simulink model "sdm_new"  (Simulink 8.1)
settings: Solver=ode45  StartTime=0.0  StopTime=65535  RelTol=1e-3
values from neighbouring files (symbols this model uses):
  sdm_in = FRAC    (= 16385)    [PSD.m]
  w = 17    [PSD.m]
undefined symbols (not defined in the file or in its folder): qunt, qunt1
settings Model: Creator=amr  LastModifiedBy=amr
settings DataIOCC: SignalLoggingSaveFormat=Dataset
settings OptimizationCC: ExpressionDepthLimit=128
settings DebuggingCC: FcnCallInpInsideContextMsg=EnableAllAsError
settings GRTTargetCC: CombineOutputUpdateFcns=on  GRTInterface=off

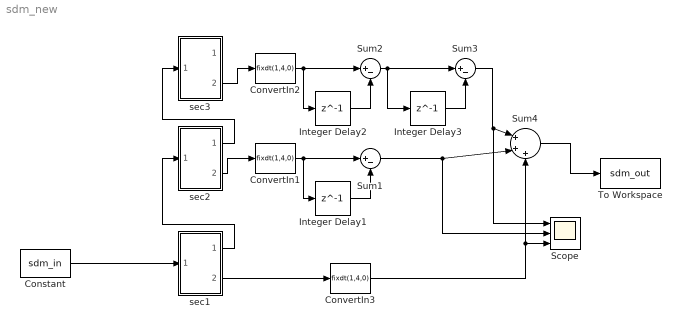
== system sdm_new ==
  Constant : Constant  Value=sdm_in  OutDataTypeStr=fixdt(1,w,0)
  ConvertIn1 : DataTypeConversion  OutDataTypeStr=fixdt(1,4,0)
  ConvertIn2 : DataTypeConversion  OutDataTypeStr=fixdt(1,4,0)
  ConvertIn3 : DataTypeConversion  OutDataTypeStr=fixdt(1,4,0)
  Integer Delay1 : Delay  DelayLength=1  InputProcessing=Inherited
  Integer Delay2 : Delay  DelayLength=1  InputProcessing=Inherited
  Integer Delay3 : Delay  DelayLength=1  InputProcessing=Inherited
  Scope : Scope  NumInputPorts=3
      settings: YMin=-1~-150000~-150000  YMax=1~150000~150000
  Sum1 : Sum  Inputs=|+-  OutDataTypeStr=fixdt(1,4,0)
  Sum2 : Sum  Inputs=|+-  OutDataTypeStr=fixdt(1,4,0)
  Sum3 : Sum  Inputs=|+-  OutDataTypeStr=fixdt(1,4,0)
  Sum4 : Sum  Inputs=|+++  OutDataTypeStr=fixdt(1,4,0)  SaturateOnIntegerOverflow=on
  To Workspace : ToWorkspace  VariableName=sdm_out  SampleTime=-1
  sec1 : Subsystem
  sec2 : Subsystem
  sec3 : Subsystem
  wires:
  Constant/1 -> sec1/1(In1)
  ConvertIn1/1 -> Integer Delay1/1, Sum1/1
  Integer Delay1/1 -> Sum1/2
  sec1/2(Out2) -> ConvertIn3/1
  Sum1/1 -> Scope/2, Sum4/2
  ConvertIn2/1 -> Integer Delay2/1, Sum2/1
  Integer Delay2/1 -> Sum2/2
  Sum2/1 -> Integer Delay3/1, Sum3/1
  Integer Delay3/1 -> Sum3/2
  Sum3/1 -> Scope/1, Sum4/1
  Sum4/1 -> To Workspace/1
  sec2/2(Out2) -> ConvertIn1/1
  sec1/1(Out1) -> sec2/1(In1)
  sec3/2(Out2) -> ConvertIn2/1
  sec2/1(Out1) -> sec3/1(In1)
  ConvertIn3/1 -> Scope/3, Sum4/3

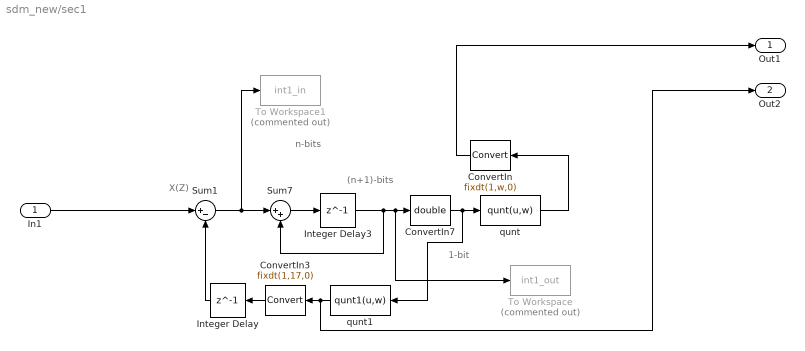
== system sdm_new/sec1 ==
  note: X(Z)
  note: 1-bit
  note: (n+1)-bits
  note: n-bits
  In1 : Inport
  ConvertIn : DataTypeConversion  OutDataTypeStr=fixdt(1,w,0)
  ConvertIn3 : DataTypeConversion  OutDataTypeStr=fixdt(1,17,0)
  ConvertIn7 : DataTypeConversion  OutDataTypeStr=double
  Integer Delay : Delay  DelayLength=1  InputProcessing=Inherited
  Integer Delay3 : Delay  DelayLength=1  InputProcessing=Inherited  SampleTime=1
  Sum1 : Sum  Inputs=|+-  OutDataTypeStr=fixdt(1,w,0)
  Sum7 : Sum  Inputs=|++  AccumDataTypeStr=fixdt(1,w+1,0)  OutDataTypeStr=fixdt(1,w+1,0)
  To Workspace : ToWorkspace  Commented=on  VariableName=int1_out  SampleTime=-1
  To Workspace1 : ToWorkspace  Commented=on  VariableName=int1_in  SampleTime=-1
  qunt : MATLABFcn  MATLABFcn=qunt(u,w)  OutputDimensions=1
  qunt1 : MATLABFcn  MATLABFcn=qunt1(u,w)  OutputDimensions=1
  Out1 : Outport
  Out2 : Outport  Port=2
  wires:
  qunt1/1 -> Out2/1, ConvertIn3/1
  Sum7/1 -> Integer Delay3/1
  qunt/1 -> ConvertIn/1
  ConvertIn7/1 -> qunt1/1, qunt/1
  Integer Delay/1 -> Sum1/2
  ConvertIn/1 -> Out1/1
  ConvertIn3/1 -> Integer Delay/1
  Sum1/1 -> To Workspace1/1, Sum7/1
  In1/1 -> Sum1/1
  Integer Delay3/1 -> To Workspace/1, ConvertIn7/1, Sum7/2

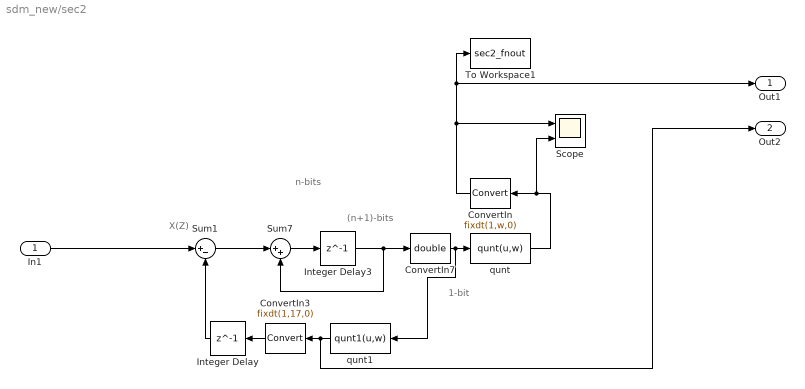
== system sdm_new/sec2 ==
  note: X(Z)
  note: 1-bit
  note: (n+1)-bits
  note: n-bits
  In1 : Inport
  ConvertIn : DataTypeConversion  OutDataTypeStr=fixdt(1,w,0)
  ConvertIn3 : DataTypeConversion  OutDataTypeStr=fixdt(1,17,0)
  ConvertIn7 : DataTypeConversion  OutDataTypeStr=double
  Integer Delay : Delay  DelayLength=1  InputProcessing=Inherited
  Integer Delay3 : Delay  DelayLength=1  InputProcessing=Inherited
  Scope : Scope  NumInputPorts=2
      settings: YMin=-70000~-140000  YMax=70000~70000
  Sum1 : Sum  Inputs=|+-  OutDataTypeStr=fixdt(1,w,0)
  Sum7 : Sum  Inputs=|++  OutDataTypeStr=fixdt(1,w+1,0)
  To Workspace1 : ToWorkspace  VariableName=sec2_fnout  SampleTime=-1
  qunt : MATLABFcn  MATLABFcn=qunt(u,w)  OutputDimensions=1
  qunt1 : MATLABFcn  MATLABFcn=qunt1(u,w)  OutputDimensions=1
  Out1 : Outport
  Out2 : Outport  Port=2
  wires:
  qunt1/1 -> Out2/1, ConvertIn3/1
  Sum7/1 -> Integer Delay3/1
  qunt/1 -> Scope/2, ConvertIn/1
  ConvertIn7/1 -> qunt1/1, qunt/1
  Integer Delay/1 -> Sum1/2
  ConvertIn/1 -> Scope/1, To Workspace1/1, Out1/1
  ConvertIn3/1 -> Integer Delay/1
  Sum1/1 -> Sum7/1
  In1/1 -> Sum1/1
  Integer Delay3/1 -> Sum7/2, ConvertIn7/1

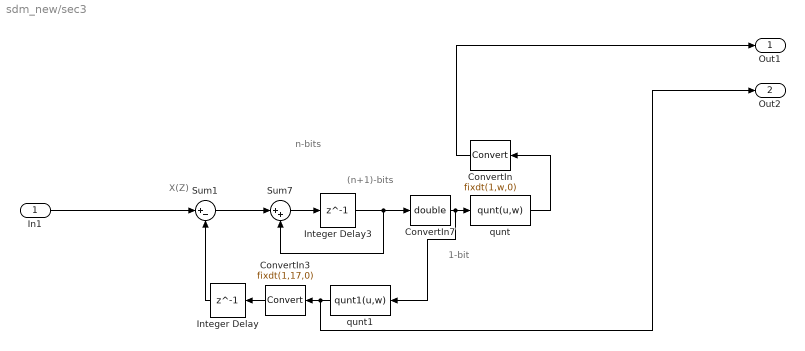
== system sdm_new/sec3 ==
  note: X(Z)
  note: 1-bit
  note: (n+1)-bits
  note: n-bits
  In1 : Inport
  ConvertIn : DataTypeConversion  OutDataTypeStr=fixdt(1,w,0)
  ConvertIn3 : DataTypeConversion  OutDataTypeStr=fixdt(1,17,0)
  ConvertIn7 : DataTypeConversion  OutDataTypeStr=double
  Integer Delay : Delay  DelayLength=1  InputProcessing=Inherited
  Integer Delay3 : Delay  DelayLength=1  InputProcessing=Inherited
  Sum1 : Sum  Inputs=|+-  OutDataTypeStr=fixdt(1,w,0)
  Sum7 : Sum  Inputs=|++  OutDataTypeStr=fixdt(1,w+1,0)
  qunt : MATLABFcn  MATLABFcn=qunt(u,w)  OutputDimensions=1
  qunt1 : MATLABFcn  MATLABFcn=qunt1(u,w)  OutputDimensions=1
  Out1 : Outport
  Out2 : Outport  Port=2
  wires:
  qunt1/1 -> Out2/1, ConvertIn3/1
  Sum7/1 -> Integer Delay3/1
  qunt/1 -> ConvertIn/1
  ConvertIn7/1 -> qunt1/1, qunt/1
  Integer Delay/1 -> Sum1/2
  ConvertIn/1 -> Out1/1
  ConvertIn3/1 -> Integer Delay/1
  Sum1/1 -> Sum7/1
  In1/1 -> Sum1/1
  Integer Delay3/1 -> Sum7/2, ConvertIn7/1
